simulink model "clik_inv"  (R2023b)
settings: Solver=ode1  StartTime=0.0  StopTime=50  FixedStep=0.001  MaxStep=0.001  RelTol=1e-6  AbsTol=1e-6
undefined symbols (not defined in the file or in its folder): DiscIntNeverNeededParam, K, q0, Tc
settings Model: Creator=fiore  LastModifiedBy=fiore
settings DataIOCC: SaveFormat=Array  SignalLoggingSaveFormat=ModelDataLogs  SaveOutput=off  SaveTime=off  ReturnWorkspaceOutputs=off
settings OptimizationCC: BlockReduction=off  BooleanDataType=off
settings DebuggingCC: SaveWithParameterizedLinksMsg=none  UnderspecifiedInitializationDetection=Classic  MergeDetectMultiDrivingBlocksExec=none  SignalResolutionControl=TryResolveAllWithWarning  MultiTaskDSMMsg=warning  MultiTaskCondExecSysMsg=none  UnconnectedInputMsg=warning  UnconnectedOutputMsg=warning  UnconnectedLineMsg=warning
settings HardwareCC: TargetUnknown=on
settings ModelReferenceCC: PropagateSignalLabelsOutOfModel=off
settings GRTTargetCC: CombineOutputUpdateFcns=off  GRTInterface=on

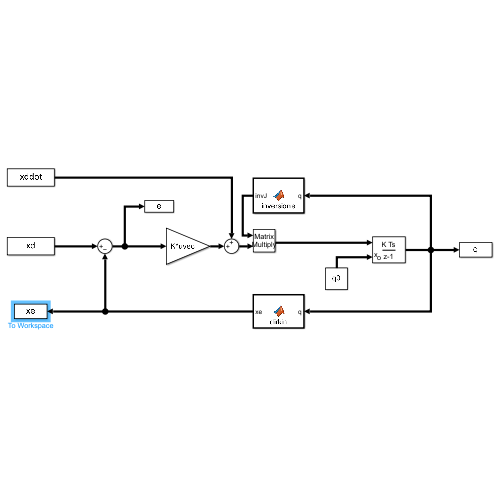
[thumbnail: Simulink's stored preview of the top-level diagram]
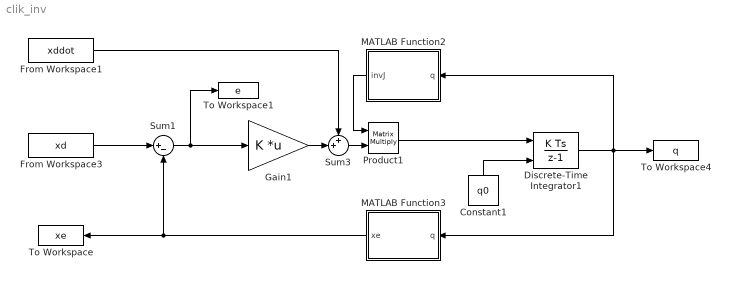
== system clik_inv ==
  Constant1 : Constant  Value=q0
  Discrete-Time Integrator1 : DiscreteIntegrator  InitialConditionSource=external  InitialCondition=q0  SampleTime=Tc  ICPrevOutput=DiscIntNeverNeededParam  ICPrevScaledInput=DiscIntNeverNeededParam
  From Workspace1 : FromWorkspace  VariableName=xddot  SampleTime=Tc
  From Workspace3 : FromWorkspace  VariableName=xd  SampleTime=Tc
  Gain1 : Gain  Gain=K  Multiplication=Matrix(K*u) (u vector)
  MATLAB Function2 : MATLAB Function  TreatAsAtomicUnit=on
  MATLAB Function3 : MATLAB Function  TreatAsAtomicUnit=on
  Product1 : Product  Multiplication=Matrix(*)
  Sum1 : Sum  Inputs=|+-
  Sum3 : Sum  Inputs=++|
  To Workspace : ToWorkspace  VariableName=xe  SaveFormat=Timeseries  SampleTime=-1
  To Workspace1 : ToWorkspace  VariableName=e  SaveFormat=Timeseries  SampleTime=-1
  To Workspace4 : ToWorkspace  VariableName=q  SaveFormat=Timeseries  SampleTime=-1
  wires:
  Product1/1 -> Discrete-Time Integrator1/1
  Sum3/1 -> Product1/2
  Discrete-Time Integrator1/1 -> MATLAB Function2/1(q), To Workspace4/1, MATLAB Function3/1(q)
  Sum1/1 -> Gain1/1, To Workspace1/1
  From Workspace3/1 -> Sum1/1
  Constant1/1 -> Discrete-Time Integrator1/2
  MATLAB Function2/1(invJ) -> Product1/1
  From Workspace1/1 -> Sum3/1
  Gain1/1 -> Sum3/2
  MATLAB Function3/1(xe) -> Sum1/2, To Workspace/1

== matlab function clik_inv/MATLAB Function3 ==
  data: q input; xe output
function xe = dirkin(q)

a1 = 0.5;
a2 = 0.5;
d0 = 1;


xe = [a1*cos(q(1))+a2*cos(q(1)+q(2));
      a1*sin(q(1))+a2*sin(q(1)+q(2));
      d0+q(3);
      q(1)+q(2)+q(4)];

end

== matlab function clik_inv/MATLAB Function2 ==
  data: invJ output; q input
function invJ=inversione(q)

a1 = 0.5;
a2 = 0.5;

J = [-a1*sin(q(1))-a2*sin(q(1)+q(2)) -a2*sin(q(1)+q(2)) 0 0;
      a1*cos(q(1))+a2*cos(q(1)+q(2))  a2*cos(q(1)+q(2)) 0 0;
                     0                         0        1 0;
                     1                         1        0 1];

invJ = pinv(J);

end
